simulink model "BSD_Warning_SWC"  (R2024a)
settings: Solver=FixedStepDiscrete  StartTime=0.0  StopTime=10.0  FixedStep=0.02  MaxStep=0.02  RelTol=1e-3
settings Model: Creator=pc  LastModifiedBy=pc
settings OptimizationCC: DefaultParameterBehavior=Inlined  EnhancedBackFolding=on  PassReuseOutputArgsAs=Individual arguments  ZeroExternalMemoryAtStartup=off  ZeroInternalMemoryAtStartup=off  OptimizeBlockOrder=speed  DifferentSizesBufferReuse=on  OptimizationCustomize=off  EfficientTunableParamExpr=on
settings DebuggingCC: ParameterTunabilityLossMsg=error
settings SFSimCC: MATLABDynamicMemAlloc=off
settings RTWCC: Description=AUTOSAR  SystemTargetFile=autosar.tlc  GenCodeOnly=on  TemplateMakefile=ert_default_tmf  DataTypeReplacement=CDataTypesFixedWidth
settings CodeAppCC: ForceParamTrailComments=on  IgnoreCustomStorageClasses=off  OperatorAnnotations=on  SimulinkDataObjDesc=on  SFDataObjDesc=on  InsertBlockDesc=on
settings STFCustomTargetCC: MultiwordLength=256  ParMdlRefBuildCompliant=on  CompOptLevelCompliant=on  IncludeMdlTerminateFcn=off  CombineOutputUpdateFcns=on  SuppressErrorStatus=on  ERTCustomFileBanners=on  SupportNonFinite=off  SupportComplex=off  SupportContinuousTime=off  SupportNonInlinedSFcns=off  RemoveResetFunc=on  MATLABClassNameForMDSCustomization=Simulink.SoftwareTarget.ERTCustomization  AutosarCompliant=on  GRTInterface=off  LookupTableObjectStructAxisOrder=2,1,3,4,...  LUTObjectStructOrderEvenSpacing=Size,Table,Breakpoints  SystemTargetFile=autosar.tlc
settings ERTTargetCC: TargetLangStandard=C99 (ISO)  ConcurrentExecutionCompliant=off  IncludeMdlTerminateFcn=off  SuppressErrorStatus=on  SupportNonFinite=off  SupportComplex=off  ModelStepFunctionPrototypeControlCompliant=off  CPPClassGenCompliant=off  AutosarCompliant=on  LookupTableObjectStructAxisOrder=2,1,3,4,...  LUTObjectStructOrderEvenSpacing=Size,Table,Breakpoints  InlinedParameterPlacement=NonHierarchical  ERTCustomFileTemplate=example_file_process.tlc  BooleanTrueId=TRUE  BooleanFalseId=FALSE

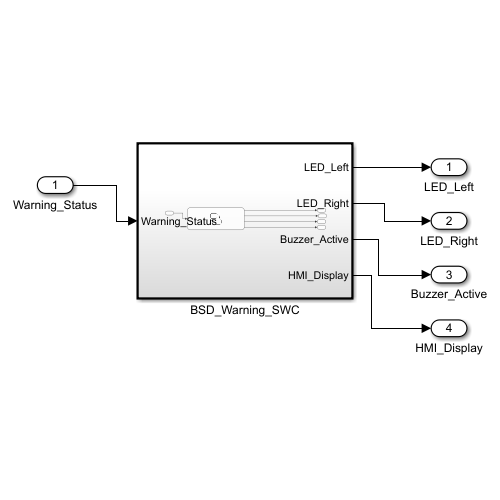
[thumbnail: Simulink's stored preview of the top-level diagram]
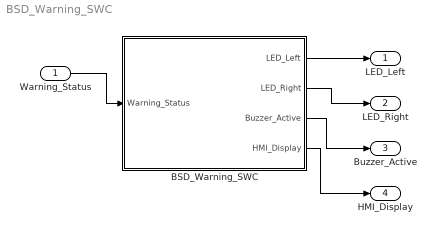
== system BSD_Warning_SWC ==
  Warning_Status : Inport  OutDataTypeStr=uint8
  BSD_Warning_SWC : Subsystem  TreatAsAtomicUnit=on  SystemSampleTime=0.02
  LED_Left : Outport  OutDataTypeStr=uint8
  LED_Right : Outport  Port=2  OutDataTypeStr=uint8
  Buzzer_Active : Outport  Port=3  OutDataTypeStr=uint8
  HMI_Display : Outport  Port=4  OutDataTypeStr=uint8
  wires:
  Warning_Status/1 -> BSD_Warning_SWC/1(Warning_Status)
  BSD_Warning_SWC/4(HMI_Display) -> HMI_Display/1
  BSD_Warning_SWC/3(Buzzer_Active) -> Buzzer_Active/1
  BSD_Warning_SWC/1(LED_Left) -> LED_Left/1
  BSD_Warning_SWC/2(LED_Right) -> LED_Right/1

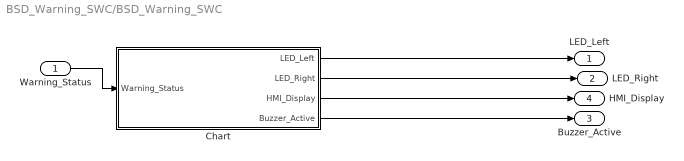
== system BSD_Warning_SWC/BSD_Warning_SWC ==
  Warning_Status : Inport
  Chart : Stateflow chart  TreatAsAtomicUnit=on
  LED_Left : Outport
  LED_Right : Outport  Port=2
  Buzzer_Active : Outport  Port=3
  HMI_Display : Outport  Port=4
  wires:
  Warning_Status/1 -> Chart/1(Warning_Status)
  Chart/4(Buzzer_Active) -> Buzzer_Active/1
  Chart/1(LED_Left) -> LED_Left/1
  Chart/2(LED_Right) -> LED_Right/1
  Chart/3(HMI_Display) -> HMI_Display/1

== stateflow chart BSD_Warning_SWC/Chart ==
  state OUTPUT_OFF
    entry:
    LED_Left      = uint8(0);
    LED_Right     = uint8(0);
    Buzzer_Active = uint8(0);
    HMI_Display   = uint8(0);
  state OUTPUT_WARNING
    entry:
    LED_Left      = uint8(1);
    LED_Right     = uint8(1);
    Buzzer_Active = uint8(0);
    HMI_Display   = uint8(1);
  state OUTPUT_ALERT
    entry:
    Buzzer_Active = uint8(1);
    HMI_Display   = uint8(2);
    during:
    Flash_Counter = Flash_Counter + uint8(1);
    if Flash_Counter >= uint8(5)
    LED_Left  = uint8(1);
    LED_Right = uint8(1);
    end
    if Flash_Counter >= uint8(10)
    LED_Left      = uint8(0);
    LED_Right     = uint8(0);
    Flash_Counter = uint8(0);
    end
  (default) -> OUTPUT_OFF
  OUTPUT_OFF -> OUTPUT_WARNING : [Warning_Status == uint8(1)]
  OUTPUT_ALERT -> OUTPUT_WARNING [order 1] : [Warning_Status == uint8(1)]
  OUTPUT_WARNING -> OUTPUT_OFF [order 1] : [Warning_Status == uint8(0)]
  OUTPUT_ALERT -> OUTPUT_OFF [order 2] : [Warning_Status == uint8(0)]
  OUTPUT_WARNING -> OUTPUT_ALERT [order 2] : [Warning_Status == uint8(2)]
  data: LED_Left output uint8 =0; LED_Right output uint8 =0; HMI_Display output uint8 =0; Buzzer_Active output uint8 =0; Warning_Status input uint8; Flash_Counter local uint8 =0
